simulink model "socEstimation"  (R2017b)
settings: Solver=VariableStepAuto  StartTime=0.0  StopTime=20000  RelTol=1e-3
PreLoadFcn:
  | socEstimation_ini
  | load('BatteryParameters')
undefined symbols (not defined in the file or in its folder): Battery, LowerSOC, sigbuilder_block, Ts, UpperSOC
libraries: fl_lib x7, nesl_utility x6, simulink x3, elec_lib x1, sharedTrackingLibrary x1
settings Model: Creator=The MathWorks, Inc.  LastModifiedBy=proso
settings DataIOCC: SignalLogging=off  DSMLogging=off  ReturnWorkspaceOutputs=on
settings OptimizationCC: DefaultParameterBehavior=Inlined  EnhancedBackFolding=on  PassReuseOutputArgsAs=Individual arguments  OptimizeBlockOrder=speed  DifferentSizesBufferReuse=on
settings DebuggingCC: ParameterTunabilityLossMsg=error
settings SFSimCC: MATLABDynamicMemAlloc=off
settings RTWCC: SystemTargetFile=ert.tlc  GenCodeOnly=on  TemplateMakefile=ert_default_tmf  GenerateReport=on  IncludeHyperlinkInReport=on  LaunchReport=on  GenerateTraceInfo=on  GenerateTraceReport=on  GenerateTraceReportSl=on  GenerateTraceReportSf=on  GenerateTraceReportEml=on
settings CodeAppCC: ForceParamTrailComments=on  IgnoreCustomStorageClasses=off  OperatorAnnotations=on  SimulinkDataObjDesc=on  SFDataObjDesc=on  InsertBlockDesc=on
settings ERTTargetCC: TargetLangStandard=C99 (ISO)  GenerateSampleERTMain=on  InlinedParameterPlacement=NonHierarchical  ERTCustomFileTemplate=example_file_process.tlc
settings SimscapeCC: SimscapeNormalizeSystem=off

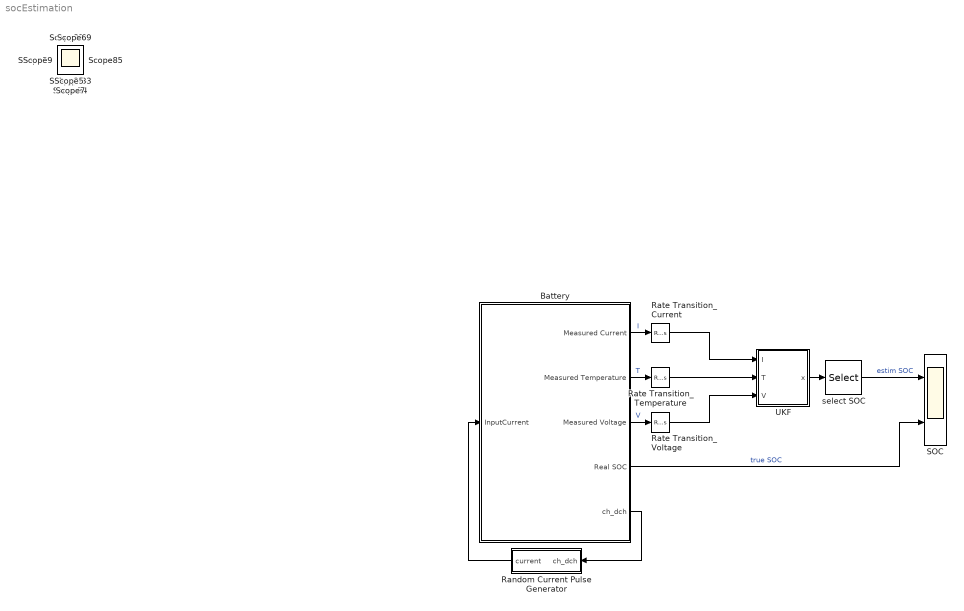
== system socEstimation ==
  Battery : Subsystem
  Random Current Pulse Generator : Subsystem
  Rate Transition_Current : RateTransition  OutPortSampleTime=Ts
  Rate Transition_Temperature : RateTransition  InitialCondition=300  OutPortSampleTime=Ts
  Rate Transition_Voltage : RateTransition  InitialCondition=4  OutPortSampleTime=Ts
  SOC : Scope  NumInputPorts=2
  UKF : Subsystem
  select SOC : Selector  InputPortWidth=4  IndexOptions=Index vector (dialog)  Indices=1  OutputSizes=1
  Scope{,1..11,13,17..18,20,22..35} (30 alike) : Scope
  wires:
  Battery/1(Measured Current) -> Rate Transition_Current/1  "I"
  Random Current Pulse Generator/1(current) -> Battery/1(InputCurrent)
  select SOC/1 -> SOC/1  "estim SOC"
  Battery/2(Measured Temperature) -> Rate Transition_Temperature/1  "T"
  Battery/3(Measured Voltage) -> Rate Transition_Voltage/1  "V"
  Battery/5(ch_dch) -> Random Current Pulse Generator/1(ch_dch)
  Rate Transition_Current/1 -> UKF/1(I)
  Rate Transition_Temperature/1 -> UKF/2(T)
  Rate Transition_Voltage/1 -> UKF/3(V)
  UKF/1(x) -> select SOC/1
  Battery/4(Real SOC) -> SOC/2  "true SOC"

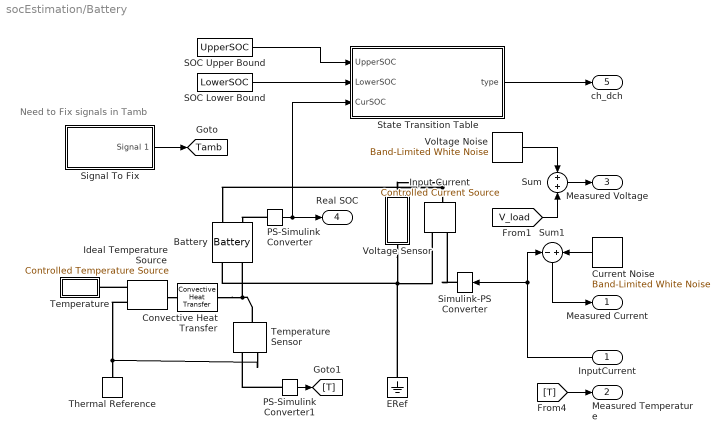
== system socEstimation/Battery ==
  note: Need to Fix signals in Tamb
  InputCurrent : Inport
  Battery : elec_lib/Sources/Battery  Vnom=3.5 V  R1=2 Ohm  prm_AH=1  AH=50 hr*A  V1=11.5 V  AH1=25 hr*A  prm_R2=1  R2=2000 Ohm  prm_fade=1  N_fade=100  AH_fade=45 hr*A  R1_fade=2.02 Ohm  V1_fade=10.35 V  i_specify=off  i_priority=None  i=0 A  i_nominal_specify=off  i_nominal_unit=A  i_nominal_value=1  v_specify=off  v_priority=None  v=0 V  v_nominal_specify=off  v_nominal_unit=V  v_nominal_value=1  charge_specify=off  charge_priority=High  charge=50 hr*A  charge_nominal_specify=off  charge_nominal_unit=hr*A  charge_nominal_value=1  num_cycles_specify=off  num_cycles_priority=High  num_cycles=0  num_cycles_nominal_specify=off  num_cycles_nominal_unit=1  num_cycles_nominal_value=1  thermal_mass=30000 J/K  Tmeas=298.15 K  Vnom_T2=3.7 V  R1_T2=2.2 Ohm  V1_T2=11.4 V  R2_T2=2200 Ohm  Tmeas2=273.15 K  temperature_specify=off  temperature_priority=High  temperature=298.15 K  temperature_nominal_specify=off  temperature_nominal_unit=K  temperature_nominal_value=1
      settings: SourceProductName=Simscape Electronics  SourceProductBaseCode=SN
  Convective Heat Transfer : fl_lib/Thermal/Thermal Elements/Convective Heat Transfer  area=cell_area m^2  heat_tr_coeff=h_conv W/(m^2 * K)  T_specify=off  T_priority=High  T=0 K  T_nominal_specify=off  T_nominal_unit=K  T_nominal_value=1  Q_specify=off  Q_priority=High  Q=0 J/s  Q_nominal_specify=off  Q_nominal_unit=J/s  Q_nominal_value=1
  Current Noise : simulink/Sources/Band-Limited White Noise  Cov=2.5e-2  Ts=Ts  seed=[1234]
  ERef : fl_lib/Electrical/Electrical Elements/Electrical Reference
  Ideal Temperature Source : fl_lib/Thermal/Thermal Sources/Controlled Temperature Source
      settings: SourceProductName=Simscape
  Input Current : fl_lib/Electrical/Electrical Sources/Controlled Current Source
  PS-Simulink Converter : nesl_utility/PS-Simulink Converter  PhysicalDomain=network_engine_domain  SubClassName=ps_output  LeftPortType=input  RightPortType=output  PseudoPeriodic=off  Frequencies=[]  Unit=1  AffineConversion=off
  PS-Simulink Converter1 : nesl_utility/PS-Simulink Converter  PhysicalDomain=network_engine_domain  SubClassName=ps_output  LeftPortType=input  RightPortType=output  PseudoPeriodic=off  Frequencies=[]  Unit=K  AffineConversion=off
  SOC Lower Bound : Constant  Value=LowerSOC
  SOC Upper Bound : Constant  Value=UpperSOC
  Signal To Fix : Subsystem  Tag=STV Subsys  LoadFcn=sigbuilder_block('load');  StartFcn=sigbuilder_block('start');  StopFcn=sigbuilder_block('stop');  ClipboardFcn=sigbuilder_block('clipboard');  mask(Sigbuilder block){tuvar=[0:10]}
      mask help: Simulink:masks:SigbuilderBlock_MD
      mask init:
      | if ~strcmp(get_param(bdroot(gcbh),'SimulationStatus'),'stopped') tuvar = sigbuilder_block('maskInit'); end
      settings: CopyFcn=sigbuilder_block('copy');  DeleteFcn=sigbuilder_block('delete');  ModelCloseFcn=sigbuilder_block('modelClose');  PreSaveFcn=sigbuilder_block('preSave');  PauseFcn=sigbuilder_block('pause');  ContinueFcn=sigbuilder_block('continue');  NameChangeFcn=sigbuilder_block('namechange');  OpenFcn=sigbuilder_block('open',[436.5 80.25 550.5 359.25 ]);  CloseFcn=sigbuilder_block('close');
      mask Display: plot(0, 0, 100, 100,[2, 2, 32, 32, 2], [68, 8, 8, 68, 68],[32, 2], [38, 38], [32, 19, 2],[53, 60, 44], [32, 17, 17, 2],[16, 16, 31, 31]);txt = getActiveGroup(gcbh);text(2, 100, txt,'verticalAlignment', 'top');
  Simulink-PS Converter : nesl_utility/Simulink-PS Converter  PhysicalDomain=network_engine_domain  SubClassName=ps_input  LeftPortType=input  RightPortType=output  PseudoPeriodic=off  Frequencies=[]  NoiseDistribution=none  NoiseParameters=[]  Unit=A  AffineConversion=off  FilteringAndDerivatives=zero  SimscapeFilterOrder=1  InputFilterTimeConstant=.001  UdotUserProvided=1
  State Transition Table : State Transition Table  TreatAsAtomicUnit=on
  Sum : Sum
  Sum1 : Sum  Inputs=-+
  Temperature : Subsystem
      mask Display: disp('Tamb')
  Temperature Sensor : fl_lib/Thermal/Thermal Sensors/Temperature Sensor
  Thermal Reference : fl_lib/Thermal/Thermal Elements/Thermal Reference
  Voltage Sensor : Subsystem
      mask Display: disp('V_load')
  Voltage Noise : simulink/Sources/Band-Limited White Noise  Cov=1.5e-3  Ts=Ts  seed=[1234]
  Measured Current : Outport
  Measured Temperature : Outport  Port=2
  Measured Voltage : Outport  Port=3
  Real SOC : Outport  Port=4
  ch_dch : Outport  Port=5
  tag scope: Tamb=global
  wires:
  SOC Lower Bound/1 -> State Transition Table/2(LowerSOC)
  SOC Upper Bound/1 -> State Transition Table/1(UpperSOC)
  Signal To Fix/1(Signal 1) -> [Tamb]
  State Transition Table/1(type) -> ch_dch/1
  [V_load] -> Sum/2
  Sum/1 -> Measured Voltage/1
  Voltage Noise/1 -> Sum/1
  Sum1/1 -> Measured Current/1
  InputCurrent/1 -> Sum1/1, Simulink-PS Converter/1
  Current Noise/1 -> Sum1/2
  [T] -> Measured Temperature/1
  PS-Simulink Converter/1 -> State Transition Table/3(CurSOC), Real SOC/1
  PS-Simulink Converter1/1 -> [T]
  connections:
  Convective Heat Transfer/RConn1 -- Temperature Sensor/LConn1 -- Battery/RConn2
  Voltage Sensor/RConn1 -- Battery/RConn1 -- Input Current/RConn2 -- ERef/LConn1
  Input Current/LConn1 -- Battery/LConn1 -- Voltage Sensor/LConn1
  Ideal Temperature Source/RConn1 -- Temperature/LConn1
  Ideal Temperature Source/RConn2 -- Thermal Reference/LConn1 -- Temperature Sensor/RConn1
  Simulink-PS Converter/RConn1 -- Input Current/RConn1
  Ideal Temperature Source/LConn1 -- Convective Heat Transfer/LConn1
  PS-Simulink Converter/LConn1 -- Battery/LConn2
  PS-Simulink Converter1/LConn1 -- Temperature Sensor/RConn2

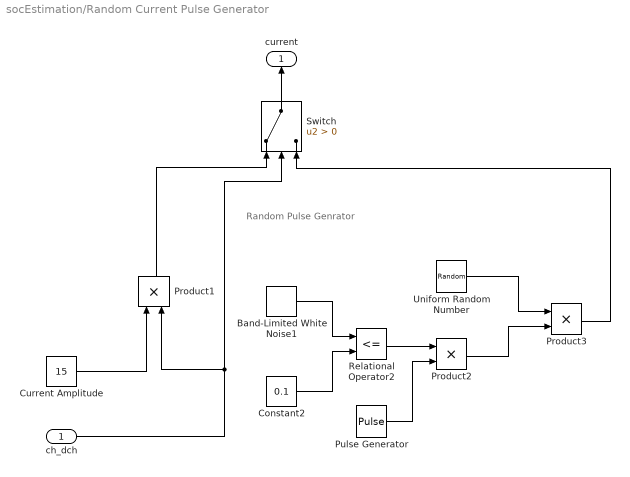
== system socEstimation/Random Current Pulse Generator ==
  note: Random Pulse Genrator
  ch_dch : Inport
  Band-Limited White Noise1 : simulink/Sources/Band-Limited White Noise  Cov=1  Ts=50  seed=[23341]
  Constant2 : Constant  Value=0.1
  Current Amplitude : Constant  Value=15
  Product1 : Product
  Product2 : Product
  Product3 : Product
  Pulse Generator : DiscretePulseGenerator  PulseType=Time based  Amplitude=-1  Period=1000  PulseWidth=90
  Relational Operator2 : RelationalOperator  Operator=<=  OutDataTypeStr=boolean  RndMeth=Simplest
  Switch : Switch  Criteria=u2 > Threshold
  Uniform Random Number : UniformRandomNumber  Minimum=5  Maximum=50  SampleTime=100
  current : Outport
  wires:
  ch_dch/1 -> Product1/2, Switch/2
  Constant2/1 -> Relational Operator2/2
  Band-Limited White Noise1/1 -> Relational Operator2/1
  Pulse Generator/1 -> Product2/2
  Relational Operator2/1 -> Product2/1
  Uniform Random Number/1 -> Product3/1
  Product2/1 -> Product3/2
  Product1/1 -> Switch/1
  Current Amplitude/1 -> Product1/1
  Product3/1 -> Switch/3
  Switch/1 -> current/1

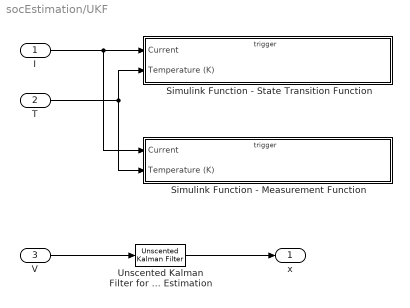
== system socEstimation/UKF ==
  I : Inport
  T : Inport  Port=2
  V : Inport  Port=3
  Simulink Function - Measurement Function : Subsystem  TreatAsAtomicUnit=on
  Simulink Function - State Transition Function : Subsystem  TreatAsAtomicUnit=on
  Unscented Kalman Filter for SOC Estimation : sharedTrackingLibrary/Unscented Kalman Filter  StateTransitionFcn=batteryStateFcn  HasAdditiveProcessNoise=Additive  ProcessNoise=1e-10*eye(4)  HasTimeVaryingProcessNoise=off  HasStateTransitionFcnExtraArgument=0  InitialState=[0.6; 0; 0; 0]  InitialStateCovariance=[1e-2 1 1 1]  Alpha=1  Beta=2  Kappa=0  MeasurementFcn1=batteryMeasurementFcn  HasMeasurementEnablePort1=off  HasAdditiveMeasurementNoise1=Additive  MeasurementNoise1=0.5  HasTimeVaryingMeasurementNoise1=off  HasMeasurementFcnExtraArgument1=0  MeasurementFcn2=myMeasurementFcn  HasMeasurementEnablePort2=off  HasAdditiveMeasurementNoise2=Additive  MeasurementNoise2=1  HasTimeVaryingMeasurementNoise2=off  HasMeasurementFcnExtraArgument2=0  MeasurementFcn3=myMeasurementFcn  HasMeasurementEnablePort3=off  HasAdditiveMeasurementNoise3=Additive  MeasurementNoise3=1  HasTimeVaryingMeasurementNoise3=off  HasMeasurementFcnExtraArgument3=0  MeasurementFcn4=myMeasurementFcn  HasMeasurementEnablePort4=off  HasAdditiveMeasurementNoise4=Additive  MeasurementNoise4=1  HasTimeVaryingMeasurementNoise4=off  HasMeasurementFcnExtraArgument4=0  MeasurementFcn5=myMeasurementFcn  HasMeasurementEnablePort5=off  HasAdditiveMeasurementNoise5=Additive  MeasurementNoise5=1  HasTimeVaryingMeasurementNoise5=off  HasMeasurementFcnExtraArgument5=0  EnableMultirate=off  StateTransitionFcnSampleTime=-1  MeasurementFcn1SampleTime=-1  MeasurementFcn2SampleTime=-1  MeasurementFcn3SampleTime=-1  MeasurementFcn4SampleTime=-1  MeasurementFcn5SampleTime=-1  UseCurrentEstimator=on  OutputStateCovariance=off  DataType=double  SampleTime=Ts  NumberOfMeasurements=1
      settings: SourceProductName=Control System Toolbox  SourceProductBaseCode=CT
  x : Outport
  wires:
  T/1 -> Simulink Function - Measurement Function/2(Temperature (K)), Simulink Function - State Transition Function/2(Temperature (K))
  V/1 -> Unscented Kalman Filter for SOC Estimation/1
  I/1 -> Simulink Function - Measurement Function/1(Current), Simulink Function - State Transition Function/1(Current)
  Unscented Kalman Filter for SOC Estimation/1 -> x/1

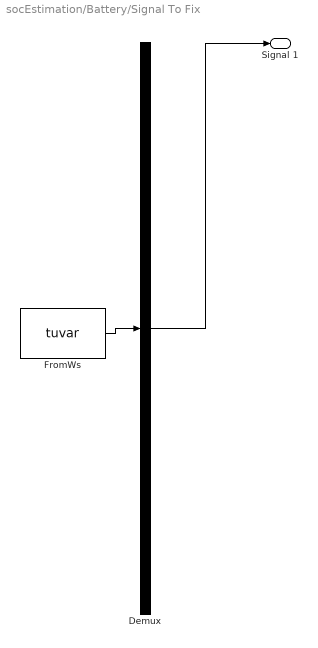
== system socEstimation/Battery/Signal To Fix ==
  Demux : Demux  Tag=STV Demux  Outputs=1
  FromWs : FromWorkspace  Tag=STV FromWs  VariableName=tuvar  SampleTime=0
      SigBuilderData=|
      | common.afterFinalStr = 'Extrapolate'
      | common.sampleTime = 0
      | dataSet.timeRange = [0 20000]
      | dataSet.name = 'Ambient Temp'
      | sbobj.Groups.Name = 'Ambient Temp'
      | sbobj.Groups.Signals.Name = 'Signal 1'
      | sbobj.Groups.Signals.XData = [0 3.8 1000 20000]
      | sbobj.Groups.Signals.YData = [0 0 50 0]
      | sbobj.Groups.TimeRange = [0 20000]
  Signal 1 : Outport  Tag=STV Outport
  wires:
  Demux/1 -> Signal 1/1
  FromWs/1 -> Demux/1

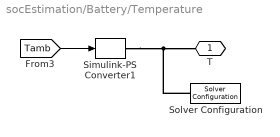
== system socEstimation/Battery/Temperature ==
  Simulink-PS Converter1 : nesl_utility/Simulink-PS Converter  PhysicalDomain=network_engine_domain  SubClassName=ps_input  LeftPortType=input  RightPortType=output  PseudoPeriodic=off  Frequencies=[]  NoiseDistribution=none  NoiseParameters=[]  Unit=degC  AffineConversion=on  FilteringAndDerivatives=zero  SimscapeFilterOrder=1  InputFilterTimeConstant=.001  UdotUserProvided=1
  Solver Configuration : nesl_utility/Solver Configuration  PhysicalDomain=network_engine_domain  SubClassName=solver  LeftPortType=input  RightPortType=generic  Accelerate=off  Tones=[]  Harmonics=[]  SimulateNoise=off  Profile=off  UseLocalSampling=off  EnableSwitchedLinearOptims=on  FrequencyDomain=off  UseCCode=off  RelTol=0.001  AbsTol=1e-06  MinStep=1e-09  ToWorkspace=off  RevertToSquareIcSolve=off  NumHomotopyIterations=100  PhasorMode=off  PhasorModeNumHarmonics=1  DoDC=off  ResidualTolerance=1e-9  UseLocalSolver=off  LocalSolverChoice=NE_BACKWARD_EULER_ADVANCER  LocalSolverSampleTime=1  DoFixedCost=off  MaxNonlinIter=3  MaxModeIter=2  LinearAlgebra=Sparse  DelaysMemoryBudget=1024  AutomaticFiltering=on  FilteringTimeConstant=0.001
  T : PMIOPort  Port=1  Side=Left
  wires:
  [Tamb] -> Simulink-PS Converter1/1
  connections:
  Simulink-PS Converter1/RConn1 -- Solver Configuration/RConn1 -- T/RConn1

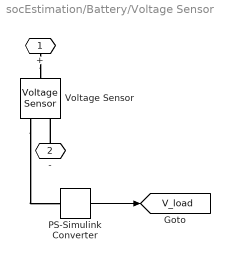
== system socEstimation/Battery/Voltage Sensor ==
  PS-Simulink Converter : nesl_utility/PS-Simulink Converter  PhysicalDomain=network_engine_domain  SubClassName=ps_output  LeftPortType=input  RightPortType=output  PseudoPeriodic=off  Frequencies=[]  Unit=V  AffineConversion=off
  Voltage Sensor : fl_lib/Electrical/Electrical Sensors/Voltage Sensor
  + : PMIOPort  Port=1  Side=Left
  - : PMIOPort  Port=2  Side=Right
  tag scope: V_load=global
  wires:
  PS-Simulink Converter/1 -> [V_load]
  connections:
  Voltage Sensor/RConn1 -- PS-Simulink Converter/LConn1
  +/RConn1 -- Voltage Sensor/LConn1
  -/RConn1 -- Voltage Sensor/RConn2

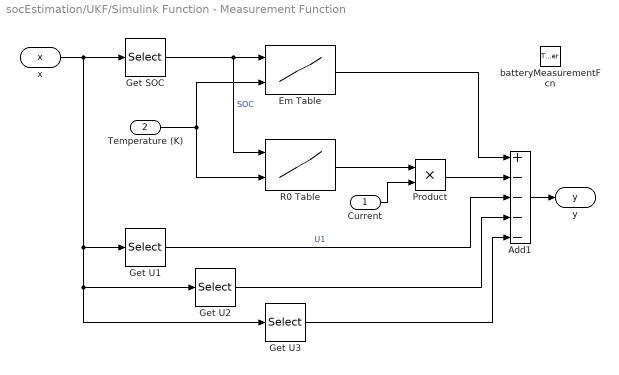
== system socEstimation/UKF/Simulink Function - Measurement Function ==
  Current : Inport
  Temperature (K) : Inport  Port=2
  batteryMeasurementFcn : TriggerPort  TriggerType=function-call  IsSimulinkFunction=on  FunctionName=batteryMeasurementFcn  VariantControl=Variant
  Add1 : Sum  Inputs=+----
  Em Table : Lookup_n-D  BreakpointsForDimension1=Battery.SOC_LUT  BreakpointsForDimension2=Battery.Temperature_LUT  Table=Battery.Em_LUT  InternalRulePriority=Speed  RndMeth=Simplest  InputSameDT=on
  Get SOC : Selector  InputPortWidth=4  IndexOptions=Index vector (dialog)  Indices=[1]  OutputSizes=1
  Get U1 : Selector  InputPortWidth=4  IndexOptions=Index vector (dialog)  Indices=2  OutputSizes=1
  Get U2 : Selector  InputPortWidth=4  IndexOptions=Index vector (dialog)  Indices=3  OutputSizes=1
  Get U3 : Selector  InputPortWidth=4  IndexOptions=Index vector (dialog)  Indices=4  OutputSizes=1
  Product : Product
  R0 Table : Lookup_n-D  BreakpointsForDimension1=Battery.SOC_LUT  BreakpointsForDimension2=Battery.Temperature_LUT  Table=Battery.R0_LUT  InternalRulePriority=Speed  RndMeth=Simplest  InputSameDT=on
  x : ArgIn  DisableCoverage=on  PortDimensions=4  ArgumentName=x
  y : ArgOut  DisableCoverage=on  ArgumentName=y
  wires:
  x/1 -> Get U3/1, Get U2/1, Get U1/1, Get SOC/1
  Get SOC/1 -> R0 Table/1, Em Table/1  "SOC"
  Em Table/1 -> Add1/1
  Add1/1 -> y/1
  Temperature (K)/1 -> R0 Table/2, Em Table/2
  R0 Table/1 -> Product/1
  Current/1 -> Product/2
  Product/1 -> Add1/2
  Get U1/1 -> Add1/3  "U1"
  Get U2/1 -> Add1/4
  Get U3/1 -> Add1/5

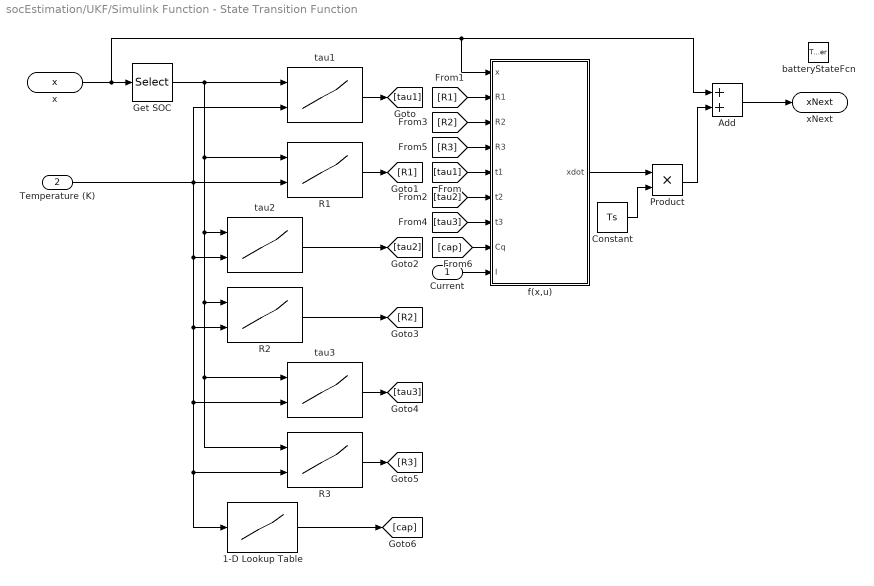
== system socEstimation/UKF/Simulink Function - State Transition Function ==
  Current : Inport
  Temperature (K) : Inport  Port=2
  batteryStateFcn : TriggerPort  TriggerType=function-call  IsSimulinkFunction=on  FunctionName=batteryStateFcn  VariantControl=Variant
  1-D Lookup Table : Lookup_n-D  NumberOfTableDimensions=1  BreakpointsForDimension1=Battery.Temperature_LUT  Table=Battery.Capacity_LUT  InternalRulePriority=Speed  RndMeth=Simplest  InputSameDT=on
  Add : Sum
  Constant : Constant  Value=Ts
  Get SOC : Selector  InputPortWidth=4  IndexOptions=Index vector (dialog)  Indices=1  OutputSizes=1
  Product : Product
  R1 : Lookup_n-D  BreakpointsForDimension1=Battery.SOC_LUT  BreakpointsForDimension2=Battery.Temperature_LUT  Table=Battery.R1_LUT  InternalRulePriority=Speed  RndMeth=Simplest  InputSameDT=on
  R2 : Lookup_n-D  BreakpointsForDimension1=Battery.SOC_LUT  BreakpointsForDimension2=Battery.Temperature_LUT  Table=Battery.R2_LUT  InternalRulePriority=Speed  RndMeth=Simplest  InputSameDT=on
  R3 : Lookup_n-D  BreakpointsForDimension1=Battery.SOC_LUT  BreakpointsForDimension2=Battery.Temperature_LUT  Table=Battery.R3_LUT  InternalRulePriority=Speed  RndMeth=Simplest  InputSameDT=on
  f(x,u) : MATLAB Function  TreatAsAtomicUnit=on
  tau1 : Lookup_n-D  BreakpointsForDimension1=Battery.SOC_LUT  BreakpointsForDimension2=Battery.Temperature_LUT  Table=Battery.t1_LUT  InternalRulePriority=Speed  RndMeth=Simplest  InputSameDT=on
  tau2 : Lookup_n-D  BreakpointsForDimension1=Battery.SOC_LUT  BreakpointsForDimension2=Battery.Temperature_LUT  Table=Battery.t2_LUT  InternalRulePriority=Speed  RndMeth=Simplest  InputSameDT=on
  tau3 : Lookup_n-D  BreakpointsForDimension1=Battery.SOC_LUT  BreakpointsForDimension2=Battery.Temperature_LUT  Table=Battery.t3_LUT  InternalRulePriority=Speed  RndMeth=Simplest  InputSameDT=on
  x : ArgIn  DisableCoverage=on  PortDimensions=4  ArgumentName=x
  xNext : ArgOut  DisableCoverage=on  PortDimensions=4  ArgumentName=xNext
  wires:
  x/1 -> f(x,u)/1(x), Add/1, Get SOC/1
  Add/1 -> xNext/1
  Temperature (K)/1 -> 1-D Lookup Table/1, R3/2, tau3/2, R2/2, tau2/2, R1/2, tau1/2
  Get SOC/1 -> R1/1, R3/1, tau3/1, R2/1, tau2/1, tau1/1
  Constant/1 -> Product/2
  f(x,u)/1(xdot) -> Product/1
  Product/1 -> Add/2
  tau1/1 -> [tau1]
  [tau1] -> f(x,u)/5(t1)
  R1/1 -> [R1]
  [R1] -> f(x,u)/2(R1)
  tau2/1 -> [tau2]
  [tau2] -> f(x,u)/6(t2)
  R2/1 -> [R2]
  [R2] -> f(x,u)/3(R2)
  R3/1 -> [R3]
  tau3/1 -> [tau3]
  [tau3] -> f(x,u)/7(t3)
  [R3] -> f(x,u)/4(R3)
  Current/1 -> f(x,u)/9(I)
  1-D Lookup Table/1 -> [cap]
  [cap] -> f(x,u)/8(Cq)

== matlab function socEstimation/UKF/Simulink Function - State Transition Function/f(x,u) ==
  data: x input; R1 input; R2 input; R3 input; t1 input; t2 input; t3 input; Cq input; I input; xdot output
function xdot = fx(x,R1,R2,R3,t1,t2,t3,Cq,I)
xdot = zeros(size(x));
U1 = x(2);
U2 = x(3);
U3 = x(4);
xdot(1) = -I/(3600*Cq);
xdot(2) = -1/t1*U1 + I/(t1/R1);
xdot(3) = -1/t2*U2 + I/(t2/R2);
xdot(4) = -1/t3*U3 + I/(t3/R3);

== stateflow chart socEstimation/Battery/State Transition Table ==
  settings: stateMachineType=MOORE_MACHINE
  state Discharge
    type = -1.0;
  state Charge
    type = 1.0;
  (default) -> Discharge
  Discharge -> (junction 166) [order 1] : [CurSOC>LowerSOC]
  (junction 166) -> Discharge
  Discharge -> Charge [order 2]
  Charge -> Discharge [order 2]
  Charge -> (junction 170) [order 1] : [CurSOC<UpperSOC]
  (junction 170) -> Charge
  data: type output =-1; UpperSOC input; LowerSOC input; CurSOC input
